simulink model "pendcart"  (Simulink 3.00)
settings: Solver=ode45  StartTime=0.0  StopTime=10.0  RelTol=1e-3
values from neighbouring files (symbols this model uses):
  g = 9.81    [cannonballpar.m]    (also in pendcartpar.m = 1; pendragpar.m)
  l = 1    [pend4par.m]    (also in pendcartpar.m; pendragpar.m = 0.1)
  m = 1    [cannonballpar.m]    (also in pendcartpar.m; pendragpar.m = 0.01)
  M = 1    [pendcartpar.m]
settings Model: SaveState=on  SaveOutput=off

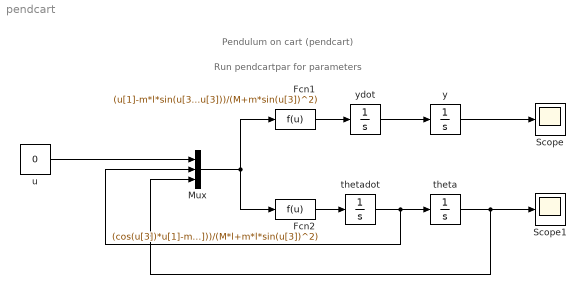
== system pendcart ==
  note: Pendulum on cart (pendcart)
  note: Run pendcartpar for parameters
  Fcn1 : Fcn  Expr=(u[1]-m*l*sin(u[3])*u[2]*u[2]-m*g*sin(u[3])*cos(u[3]))/(M+m*sin(u[3])^2)
  Fcn2 : Fcn  Expr=(cos(u[3])*u[1]-m*l*sin(u[3])*cos(u[3])*u[2]*u[2]-(M+m)*g*sin(u[3]))/(M*l+m*l*sin(u[3])^2)
  Mux : Mux  Inputs=3
  Scope : Scope
      settings: TimeRange=auto  YMin=-5  YMax=5  SaveToWorkspace=off  SaveName=ScopeData
  Scope1 : Scope
      settings: TimeRange=auto  YMin=-5  YMax=5  SaveToWorkspace=off  SaveName=ScopeData
  theta : Integrator  ExternalReset=none  InitialConditionSource=internal  InitialCondition=pi/2  LimitOutput=off  UpperSaturationLimit=inf  LowerSaturationLimit=-inf  ShowSaturationPort=off  ShowStatePort=off  AbsoluteTolerance=auto
  thetadot : Integrator  ExternalReset=none  InitialConditionSource=internal  InitialCondition=0  LimitOutput=off  UpperSaturationLimit=inf  LowerSaturationLimit=-inf  ShowSaturationPort=off  ShowStatePort=off  AbsoluteTolerance=auto
  u : Constant  Value=0
  y : Integrator  ExternalReset=none  InitialConditionSource=internal  InitialCondition=0  LimitOutput=off  UpperSaturationLimit=inf  LowerSaturationLimit=-inf  ShowSaturationPort=off  ShowStatePort=off  AbsoluteTolerance=auto
  ydot : Integrator  ExternalReset=none  InitialConditionSource=internal  InitialCondition=0  LimitOutput=off  UpperSaturationLimit=inf  LowerSaturationLimit=-inf  ShowSaturationPort=off  ShowStatePort=off  AbsoluteTolerance=auto
  wires:
  Mux/1 -> Fcn1/1, Fcn2/1
  Fcn2/1 -> thetadot/1
  Fcn1/1 -> ydot/1
  thetadot/1 -> theta/1, Mux/2
  theta/1 -> Scope1/1, Mux/3
  y/1 -> Scope/1
  u/1 -> Mux/1
  ydot/1 -> y/1
